simulink model "alfa147gta"  (R2017b)
settings: Solver=VariableStepAuto  StartTime=0.0  StopTime=10.0  RelTol=1e-3
PreLoadFcn:
  | load('alfa147gta.mat')
values from neighbouring files (symbols this model uses):
  EngineRPM = [1000 1500 2000 2500 3000 3500 4000 4500 5000 5500 6000 6500 ... (13 elements, 1x13)]    [alfa147gta.mat]    (also in cruise_control_sim.mat)
  EngineTRQ = [200 220 242 258 260 261 268 285 300 296 290 250 ... (13 elements, 1x13)]    [alfa147gta.mat]    (also in cruise_control_sim.mat)
  FinalRatio = 3.733    [alfa147gta.mat]    (also in cruise_control_sim.mat)
  GearRatio = [3.5 2.235 1.52 1.156 0.971 0.818]    [alfa147gta.mat]    (also in cruise_control_sim.mat)
  Kdrag = 0.4238432    [alfa147gta.mat]    (also in cruise_control_sim.mat)
  Mass = 1360    [alfa147gta.mat]    (also in cruise_control_sim.mat)
  WheelRadius = 0.2992    [alfa147gta.mat]    (also in cruise_control_sim.mat)
settings Model: Creator=Michele  LastModifiedBy=Michele

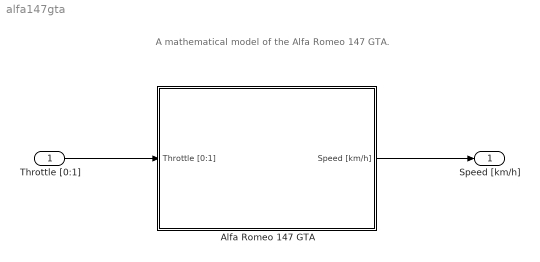
== system alfa147gta ==
  note: A mathematical model of the Alfa Romeo 147 GTA.
  Throttle [0:1] : Inport
  Alfa Romeo 147 GTA : Subsystem
  Speed [km/h] : Outport
  wires:
  Throttle [0:1]/1 -> Alfa Romeo 147 GTA/1(Throttle [0:1])
  Alfa Romeo 147 GTA/1(Speed [km/h]) -> Speed [km/h]/1

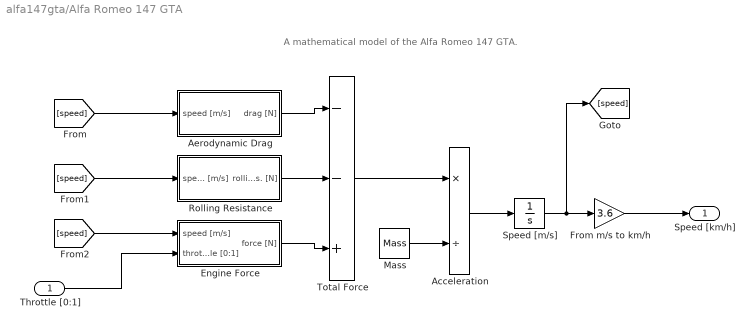
== system alfa147gta/Alfa Romeo 147 GTA ==
  note: A mathematical model of the Alfa Romeo 147 GTA.
  Throttle [0:1] : Inport
  Acceleration : Product  Inputs=*/
  Aerodynamic Drag : Subsystem
  Engine Force : Subsystem
  From m/s to km/h : Gain  Gain=3.6
  Mass : Constant  Value=Mass
  Rolling Resistance : Subsystem
  Speed [m/s] : Integrator
  Total Force : Sum  Inputs=--+
  Speed [km/h] : Outport
  wires:
  [speed] -> Aerodynamic Drag/1("speed [m/s] ")
  Aerodynamic Drag/1(drag [N]) -> Total Force/1
  Rolling Resistance/1(rolling res. [N]) -> Total Force/2
  Speed [m/s]/1 -> [speed], From m/s to km/h/1
  Engine Force/1(force [N]) -> Total Force/3
  From m/s to km/h/1 -> Speed [km/h]/1
  Mass/1 -> Acceleration/2
  Acceleration/1 -> Speed [m/s]/1
  Total Force/1 -> Acceleration/1
  Throttle [0:1]/1 -> Engine Force/2(throttle [0:1])
  [speed] -> Rolling Resistance/1(speed [m/s])
  [speed] -> Engine Force/1(speed [m/s])

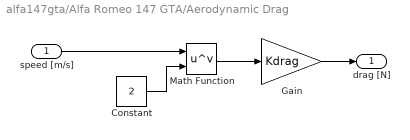
== system alfa147gta/Alfa Romeo 147 GTA/Aerodynamic Drag ==
  "speed [m/s] " : Inport
  Constant : Constant  Value=2
  Gain : Gain  Gain=Kdrag
  Math Function : Math  Operator=pow  SaturateOnIntegerOverflow=on
  drag [N] : Outport
  wires:
  "speed [m/s] "/1 -> Math Function/1
  Constant/1 -> Math Function/2
  Gain/1 -> drag [N]/1
  Math Function/1 -> Gain/1

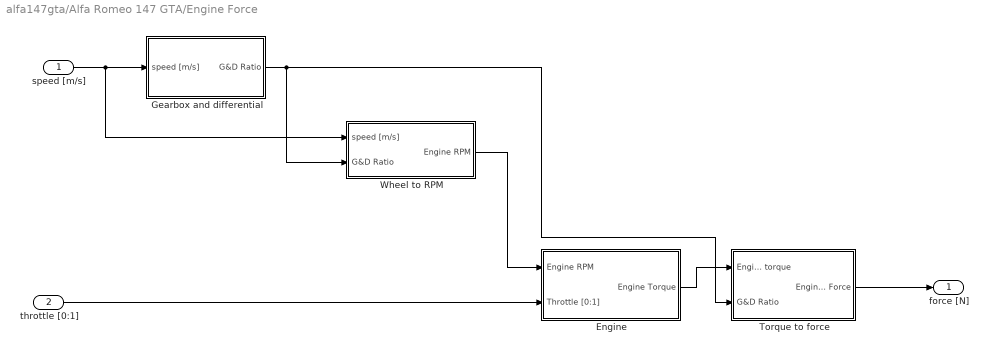
== system alfa147gta/Alfa Romeo 147 GTA/Engine Force ==
  speed [m/s] : Inport
  throttle [0:1] : Inport  Port=2
  Engine : Subsystem
  Gearbox and differential : Subsystem
  Torque to force : Subsystem
  Wheel to RPM : Subsystem
  force [N] : Outport
  wires:
  speed [m/s]/1 -> Wheel to RPM/1("speed [m/s] "), Gearbox and differential/1(speed [m/s])
  Wheel to RPM/1(Engine RPM) -> Engine/1(Engine RPM)
  Gearbox and differential/1(G&D Ratio) -> Torque to force/2(G&D Ratio), Wheel to RPM/2("G&D Ratio ")
  throttle [0:1]/1 -> Engine/2(Throttle [0:1])
  Engine/1(Engine Torque) -> Torque to force/1(Engine torque)
  Torque to force/1(Engine Force) -> force [N]/1

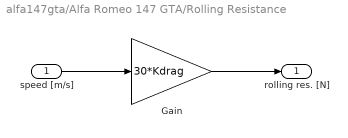
== system alfa147gta/Alfa Romeo 147 GTA/Rolling Resistance ==
  speed [m/s] : Inport
  Gain : Gain  Gain=30*Kdrag
  rolling res. [N] : Outport
  wires:
  speed [m/s]/1 -> Gain/1
  Gain/1 -> rolling res. [N]/1

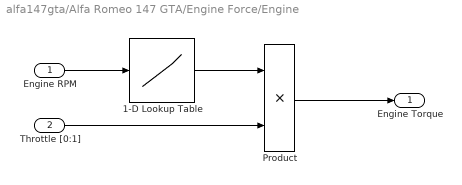
== system alfa147gta/Alfa Romeo 147 GTA/Engine Force/Engine ==
  Engine RPM : Inport
  Throttle [0:1] : Inport  Port=2
  1-D Lookup Table : Lookup_n-D  NumberOfTableDimensions=1  BreakpointsForDimension1=EngineRPM  Table=EngineTRQ  InterpMethod=Cubic spline  InternalRulePriority=Speed  RndMeth=Simplest  InputSameDT=on
  Product : Product
  Engine Torque : Outport
  wires:
  Engine RPM/1 -> 1-D Lookup Table/1
  1-D Lookup Table/1 -> Product/1
  Throttle [0:1]/1 -> Product/2
  Product/1 -> Engine Torque/1

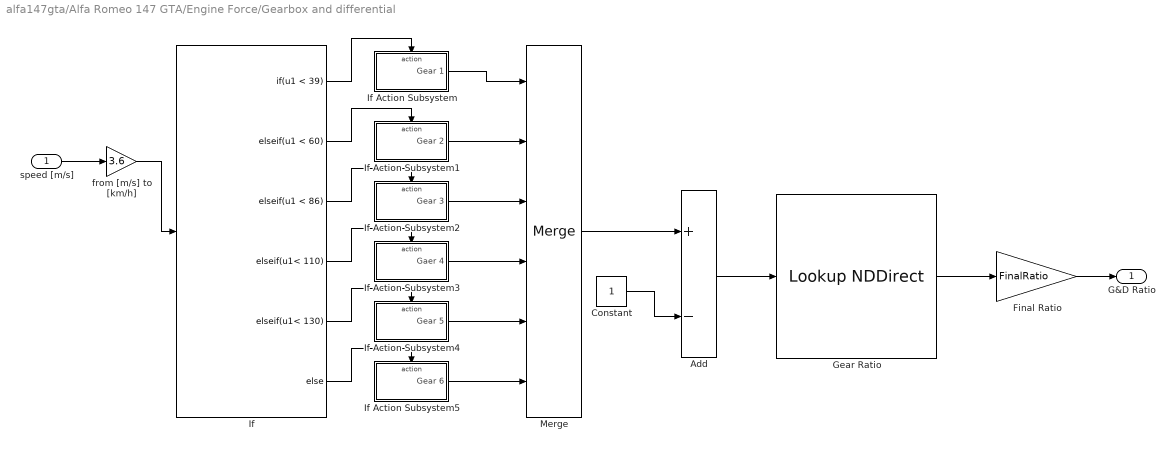
== system alfa147gta/Alfa Romeo 147 GTA/Engine Force/Gearbox and differential ==
  speed [m/s] : Inport
  Add : Sum  Inputs=+-
  Constant : Constant
  Final Ratio : Gain  Gain=FinalRatio
  Gear Ratio : LookupNDDirect  NumberOfTableDimensions=1  Table=GearRatio
  If : If  IfExpression=u1 < 39  ElseIfExpressions=u1 < 60, u1 < 86, u1< 110, u1< 130
  If Action Subsystem : Subsystem  TreatAsAtomicUnit=on
  If Action Subsystem1 : Subsystem  TreatAsAtomicUnit=on
  If Action Subsystem2 : Subsystem  TreatAsAtomicUnit=on
  If Action Subsystem3 : Subsystem  TreatAsAtomicUnit=on
  If Action Subsystem4 : Subsystem  TreatAsAtomicUnit=on
  If Action Subsystem5 : Subsystem  TreatAsAtomicUnit=on
  Merge : Merge  Inputs=6
  from [m/s] to [km/h] : Gain  Gain=3.6
  G&D Ratio : Outport
  wires:
  speed [m/s]/1 -> from [m/s] to [km/h]/1
  from [m/s] to [km/h]/1 -> If/1
  If/1 -> If Action Subsystem/Action
  If/2 -> If Action Subsystem1/Action
  If/3 -> If Action Subsystem2/Action
  If/4 -> If Action Subsystem3/Action
  If/5 -> If Action Subsystem4/Action
  If/6 -> If Action Subsystem5/Action
  If Action Subsystem/1(Gear 1) -> Merge/1
  If Action Subsystem5/1(Gear 6) -> Merge/6
  If Action Subsystem4/1(Gear 5) -> Merge/5
  If Action Subsystem3/1(Gaer 4) -> Merge/4
  If Action Subsystem2/1(Gear 3) -> Merge/3
  If Action Subsystem1/1(Gear 2) -> Merge/2
  Add/1 -> Gear Ratio/1
  Merge/1 -> Add/1
  Constant/1 -> Add/2
  Gear Ratio/1 -> Final Ratio/1
  Final Ratio/1 -> G&D Ratio/1

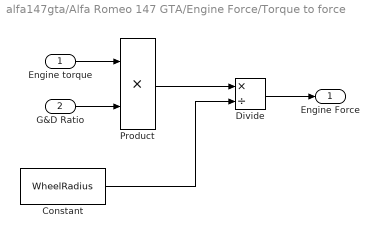
== system alfa147gta/Alfa Romeo 147 GTA/Engine Force/Torque to force ==
  Engine torque : Inport
  G&D Ratio : Inport  Port=2
  Constant : Constant  Value=WheelRadius
  Divide : Product  Inputs=*/
  Product : Product
  Engine Force : Outport
  wires:
  G&D Ratio/1 -> Product/2
  Engine torque/1 -> Product/1
  Product/1 -> Divide/1
  Constant/1 -> Divide/2
  Divide/1 -> Engine Force/1

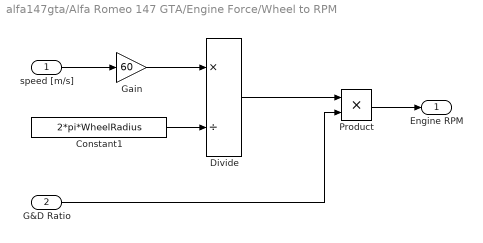
== system alfa147gta/Alfa Romeo 147 GTA/Engine Force/Wheel to RPM ==
  "speed [m/s] " : Inport
  "G&D Ratio " : Inport  Port=2
  Constant1 : Constant  Value=2*pi*WheelRadius
  Divide : Product  Inputs=*/
  Gain : Gain  Gain=60
  Product : Product
  Engine RPM : Outport
  wires:
  Gain/1 -> Divide/1
  "speed [m/s] "/1 -> Gain/1
  Constant1/1 -> Divide/2
  Divide/1 -> Product/1
  "G&D Ratio "/1 -> Product/2
  Product/1 -> Engine RPM/1

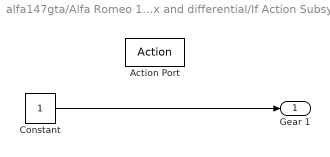
== system alfa147gta/Alfa Romeo 147 GTA/Engine Force/Gearbox and differential/If Action Subsystem ==
  Action Port : ActionPort  ActionType=then
  Constant : Constant
  Gear 1 : Outport
  wires:
  Constant/1 -> Gear 1/1

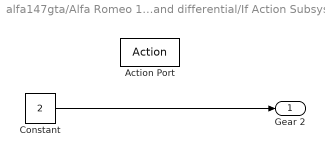
== system alfa147gta/Alfa Romeo 147 GTA/Engine Force/Gearbox and differential/If Action Subsystem1 ==
  Action Port : ActionPort  ActionType=elseif
  Constant : Constant  Value=2
  Gear 2 : Outport
  wires:
  Constant/1 -> Gear 2/1

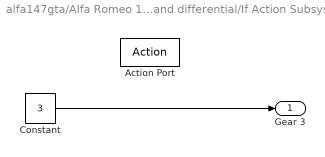
== system alfa147gta/Alfa Romeo 147 GTA/Engine Force/Gearbox and differential/If Action Subsystem2 ==
  Action Port : ActionPort  ActionType=elseif
  Constant : Constant  Value=3
  Gear 3 : Outport
  wires:
  Constant/1 -> Gear 3/1

== system alfa147gta/Alfa Romeo 147 GTA/Engine Force/Gearbox and differential/If Action Subsystem3 ==
  Action Port : ActionPort  ActionType=elseif
  Constant : Constant  Value=4
  Gaer 4 : Outport
  wires:
  Constant/1 -> Gaer 4/1

== system alfa147gta/Alfa Romeo 147 GTA/Engine Force/Gearbox and differential/If Action Subsystem4 ==
  Action Port : ActionPort  ActionType=elseif
  Constant : Constant  Value=5
  Gear 5 : Outport
  wires:
  Constant/1 -> Gear 5/1

== system alfa147gta/Alfa Romeo 147 GTA/Engine Force/Gearbox and differential/If Action Subsystem5 ==
  Action Port : ActionPort  ActionType=else
  Constant : Constant  Value=6
  Gear 6 : Outport
  wires:
  Constant/1 -> Gear 6/1
